simulink model "matlabFuncBlock_simulink"  (R2022b)
settings: Solver=VariableStepAuto  StartTime=0.0  StopTime=10.0  RelTol=1e-3
settings Model: Creator=chris  LastModifiedBy=chris
settings SFSimCC: SimCustomHeaderCode="#include \"add_lib.h\""  SimUserSources=main.c

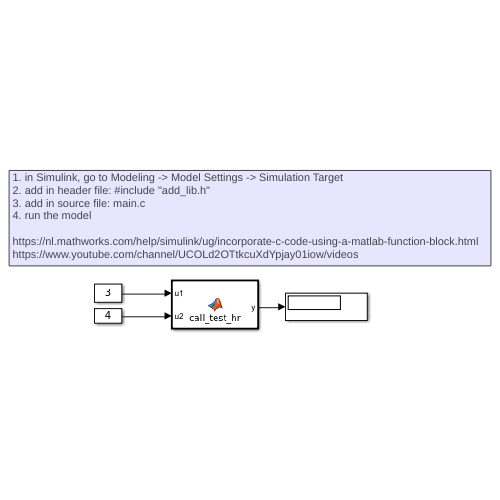
[thumbnail: Simulink's stored preview of the top-level diagram]
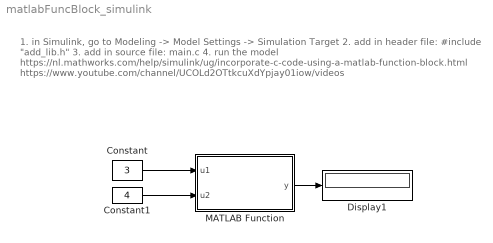
== system matlabFuncBlock_simulink ==
  note: 1. in Simulink, go to Modeling -> Model Settings -> Simulation Target
      | 2. add in header file: #include "add_lib.h"
      | 3. add in source file: main.c
      | 4. run the model
      |
      | https://nl.mathworks.com/help/simulink/ug/incorporate-c-code-using-a-matlab-function-block.html
      | https://www.youtube.com/channel/UCOLd2OTtkcuXdYpjay01iow/videos
  Constant : Constant  Value=3
  Constant1 : Constant  Value=4
  Display1 : Display
  MATLAB Function : MATLAB Function  TreatAsAtomicUnit=on
  wires:
  Constant/1 -> MATLAB Function/1(u1)
  Constant1/1 -> MATLAB Function/2(u2)
  MATLAB Function/1(y) -> Display1/1

== matlab function matlabFuncBlock_simulink/MATLAB Function ==
  data: u1 input; y output; u2 input
function y = call_test_hr(u1, u2)
%#codegen
    x = 0.0;
    x = coder.ceval('add_2',u1, u2);    
y = x;
